simulink model "mysim22"  (R2021b)
settings: Solver=ode23t  StartTime=0.0  StopTime=70  RelTol=1e-3
libraries: fl_lib x15, nesl_utility x9, simulink x9, sh_lib x3, slpidlib x2
settings Model: Creator=camil  LastModifiedBy=camil

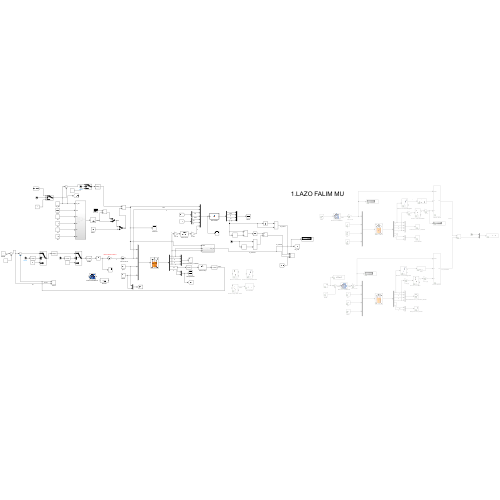
[thumbnail: Simulink's stored preview of the top-level diagram]
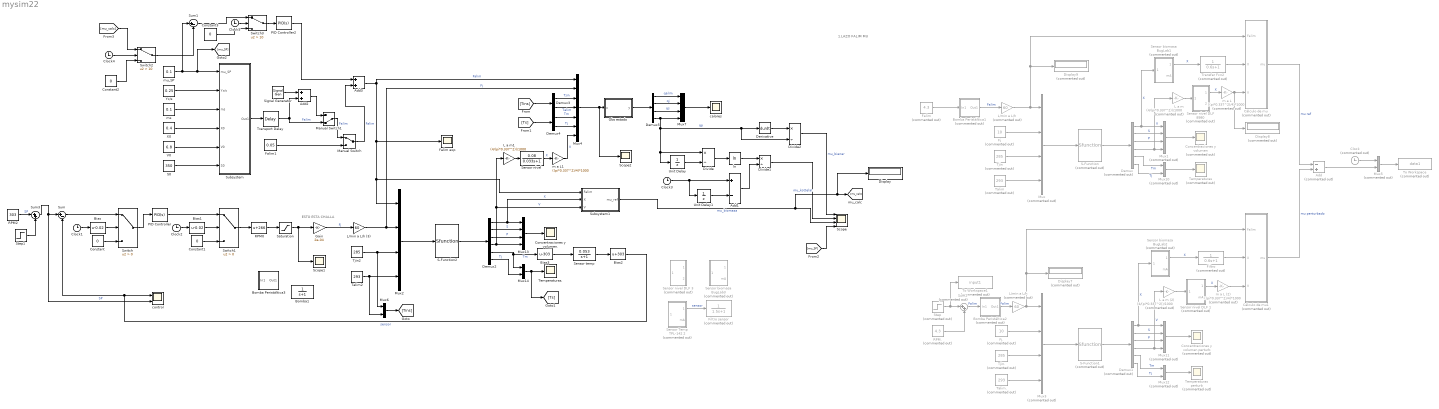
== system mysim22 ==
  note: ESTO ESTA CHALLA
  note: 1.LAZO FALIM MU
  Add : Sum  Commented=on  Inputs=-+
  Add1 : Sum  Inputs=+-
  Add2 : Sum
  Add3 : Sum
  Bias : Bias  Bias=-0.02
  Bias1 : Bias  Bias=-0.02
  Bias2 : Bias  Bias=303
  Bias3 : Bias  Bias=-303
  Bomba Peristáltica1 : Subsystem  Commented=on  mask{D=0.0002, MaxRPM=100, MaxLPM=0.036, OutP=0.14, FluidDens=997, KinemVisc=0.893e-6, BulkMod=2.2e+9}
      mask prompts: D "Displacement [L/rev]"; MaxRPM "RPM Máximas [RPM]"; MaxLPM "Caudal Máximo [L/min]"; OutP "Presión de Salida [MPa]"; FluidDens "Densidad del Fluido [kg/m^3]"; KinemVisc "Viscosidad Cinemática del Fluido [m^2/s]"; BulkMod "Modulo de Compresibilidad del Fluido [Pa]"
      mask help:
      | Simulación de una Bomba Peristáltica utilizando el paquete Simscape (puede entrar en el subsistema para ver en base a que bloques se construyó).
      |
      | El principal parámetro es el Displacement, que representa cuánto aumenta el flujo de la bomba medido en Litros por Minuto [L/min] según el aumento unitario de Revoluciones por Minuto [RPM].
      |
      | El input de este bloque es una fuente de revoluciones en unidades de RPM, el cual entrega un output de caudal en L/min.
      |
      | El valor del Displacement no puede superar su valor máximo según los parámetros entregados de la bomba.
      mask Display: image('bomba_peristaltica.jpg'); % Use "Edit Image" on toolstrip to change.
  Bomba Peristáltica2 : Subsystem  Commented=on  mask{D=0.0002, MaxRPM=100, MaxLPM=0.036, OutP=0.14, FluidDens=997, KinemVisc=0.893e-6, BulkMod=2.2e+9}
      mask prompts: D "Displacement [L/rev]"; MaxRPM "RPM Máximas [RPM]"; MaxLPM "Caudal Máximo [L/min]"; OutP "Presión de Salida [MPa]"; FluidDens "Densidad del Fluido [kg/m^3]"; KinemVisc "Viscosidad Cinemática del Fluido [m^2/s]"; BulkMod "Modulo de Compresibilidad del Fluido [Pa]"
      mask help:
      | Simulación de una Bomba Peristáltica utilizando el paquete Simscape (puede entrar en el subsistema para ver en base a que bloques se construyó).
      |
      | El principal parámetro es el Displacement, que representa cuánto aumenta el flujo de la bomba medido en Litros por Minuto [L/min] según el aumento unitario de Revoluciones por Minuto [RPM].
      |
      | El input de este bloque es una fuente de revoluciones en unidades de RPM, el cual entrega un output de caudal en L/min.
      |
      | El valor del Displacement no puede superar su valor máximo según los parámetros entregados de la bomba.
      mask Display: image('bomba_peristaltica.jpg'); % Use "Edit Image" on toolstrip to change.
  Bomba Peristáltica3 : Subsystem  mask{D=0.05, MaxRPM=330, MaxLPM=19.4, OutP=0.141, FluidDens=997, KinemVisc=0.893e-6, BulkMod=2.2e+9}
      mask prompts: D "Displacement [L/rev]"; MaxRPM "RPM Máximas [RPM]"; MaxLPM "Caudal Máximo [L/min]"; OutP "Presión de Salida [MPa]"; FluidDens "Densidad del Fluido [kg/m^3]"; KinemVisc "Viscosidad Cinemática del Fluido [m^2/s]"; BulkMod "Modulo de Compresibilidad del Fluido [Pa]"
      mask help:
      | Simulación de una Bomba Peristáltica utilizando el paquete Simscape (puede entrar en el subsistema para ver en base a que bloques se construyó).
      |
      | El principal parámetro es el Displacement, que representa cuánto aumenta el flujo de la bomba medido en Litros por Minuto [L/min] según el aumento unitario de Revoluciones por Minuto [RPM].
      |
      | El input de este bloque es una fuente de revoluciones en unidades de RPM, el cual entrega un output de caudal en L/min.
      |
      | El valor del Displacement no puede superar su valor máximo según los parámetros entregados de la bomba.
      mask Display: image('bomba_peristaltica.jpg'); % Use "Edit Image" on toolstrip to change.
  Bomba1 : TransferFcn  Denominator=[1 1]
  Clock : Clock  Commented=on
  Clock{1..5} (5 alike) : Clock
  Concentraciones y volumen : Scope  Commented=on
  Concentraciones y volumen perturb : Scope  Commented=on
  Concentraciones y volumen. : Scope
  Constant{,1..3} (4 alike) : Constant  Value=0
  Cálculo de mu : Subsystem  Commented=on
  Cálculo de mu1 : Subsystem  Commented=on
  Demux : Demux  Commented=on  Outputs=6
  Demux1 : Demux  Commented=on  Outputs=6
  Demux2 : Demux  Outputs=6
  Demux3 : Demux  Outputs=2
  Demux4 : Demux  Outputs=2
  Demux5 : Demux
  Derivative : Derivative
  Display : Display
  Display7 : Display  Commented=on
  Display8 : Display  Commented=on
  Display9 : Display  Commented=on
  Divide : Product  Inputs=*/
  Divide1 : Product  Inputs=*/
  Divide2 : Product  Inputs=*/
  Falim : Constant  Commented=on  Value=4.3
  Falim exp : Scope
  Falim1 : Constant  Value=0.05
  Filtro : TransferFcn  Commented=on  Denominator=[0.6 1]
  Filtro sensor : TransferFcn  Commented=on  Denominator=[1.5 1]
  Fj : Constant  Commented=on  Value=10
  Fj. : Constant  Commented=on  Value=10
  Gain : Gain  Gain=2e-04
  L a m : Gain  Commented=on  Gain=(4/(pi*0.337^2))/1000
  L a m (2) : Gain  Commented=on  Gain=(4/(pi*0.337^2))/1000
  L a m1 : Gain  Gain=(4/(pi*0.337^2))/1000
  L/min a L/h : Gain  Commented=on  Gain=60
  "L/min a L/h " : Gain  Commented=on  Gain=60
  L/min a L/h (3) : Gain  Gain=60
  Manual Switch : ManualSwitch
  Manual Switch1 : ManualSwitch  CurrentSetting=0
  Mux{,1,3,11} (4 alike) : Mux  Commented=on
  Mux10 : Mux  Commented=on  Inputs=2
  Mux12 : Mux  Commented=on  Inputs=2
  Mux13 : Mux
  Mux14 : Mux  Inputs=2
  Mux2 : Mux
  Mux4 : Mux  Inputs=7
  Mux5 : Mux  Commented=on  Inputs=2
  Mux6 : Mux  Inputs=2
  Mux7 : Mux
  Obs estado : MATLAB Function  TreatAsAtomicUnit=on
  PID Controller : slpidlib/PID Controller  Controller=PID  Form=Parallel  TimeDomain=Continuous-time  UseExternalTs=off  SampleTime=-1  IntegratorMethod=Forward Euler  FilterMethod=Forward Euler  ControllerParametersSource=internal  P=-2.038e+06  I=-6.635e+04  D=0  UseFilter=on  N=100  TunerSelectOption=Transfer Function Based (PID Tuner App)  InitialConditionSource=internal  InitialConditionForIntegrator=0  InitialConditionForFilter=0  DifferentiatorICPrevScaledInput=0  ExternalReset=none  TrackingMode=off  Kt=1  LimitOutput=off  SatLimitsSource=internal  UpperSaturationLimit=inf  LowerSaturationLimit=-inf  LinearizeAsGain=on  AntiWindupMode=none  Kb=1  RndMeth=Zero  POutMin=[]  POutMax=[]  IOutMin=[]  IOutMax=[]  DOutMin=[]  DOutMax=[]  NOutMin=[]  NOutMax=[]  SumOutMin=[]  SumOutMax=[]  SaturationOutMin=[]  SaturationOutMax=[]  PParamMin=[]  PParamMax=[]  IParamMin=[]  IParamMax=[]  DParamMin=[]  DParamMax=[]  NParamMin=[]  NParamMax=[]  KbParamMin=[]  KbParamMax=[]  KtParamMin=[]  KtParamMax=[]  KbOutMin=[]  KbOutMax=[]  KtOutMin=[]  KtOutMax=[]  IntegratorOutMin=[]  IntegratorOutMax=[]  FilterOutMin=[]  FilterOutMax=[]  SumI1OutMin=[]  SumI1OutMax=[]  SumI2OutMin=[]  SumI2OutMax=[]  SumI3OutMin=[]  SumI3OutMax=[]  SumI4OutMin=[]  SumI4OutMax=[]  SumDOutMin=[]  SumDOutMax=[]  DifferentiatorOutMin=[]  DifferentiatorOutMax=[]  FilterDiffOutCoefMin=[]  FilterDiffOutCoefMax=[]  ReciprocalOutMin=[]  ReciprocalOutMax=[]  SumDenOutMin=[]  SumDenOutMax=[]  SumNumOutMin=[]  SumNumOutMax=[]  DivideOutMin=[]  DivideOutMax=[]  UdiffTsProdOutMin=[]  UdiffTsProdOutMax=[]  NTsProdOutMin=[]  NTsProdOutMax=[]  UintegralTsProdOutMin=[]  UintegralTsProdOutMax=[]  UngainTsProdOutMin=[]  UngainTsProdOutMax=[]  IntegratorContinuousStateAttributes=''  IntegratorStateMustResolveToSignalObject=off  IntegratorRTWStateStorageClass=Auto  FilterContinuousStateAttributes=''  FilterStateMustResolveToSignalObject=off  FilterRTWStateStorageClass=Auto  ParallelPVariant=InternalParameters  IdealPVariant=Disabled  IVariant=InternalParameters  DVariant=InternalParameters  IntegratorVariant=Continuous  SatVariant=Disabled  AWVariant=Passthrough  PCopyVariant=Disabled  TRVariant=Disabled  FdbkBlocksVariant=Forward  IdealPFdbkVariant=Disabled  SatFdbkVariant=Disabled  DerivativeFilterVariant=ContFilter  NVariant=InternalParameters  NCopyVariant=Disabled  FilterICVariant=InternalICsFilter  IntegratorICVariant=InternalICs  ExternalResetVariant=Disabled  TRSumVariant=Passthrough  SumFdbkVariant=Disabled  SumVariant=Sum_PID  TsampFilterVariant=InternalTs  TsampNgainVariant=Passthrough  TsampIntegralVariant=Passthrough  ExternalSaturationOutDataTypeStr=Inherit: Same as second input
  PID Controller2 : slpidlib/PID Controller  Controller=PID  Form=Parallel  TimeDomain=Continuous-time  UseExternalTs=off  SampleTime=-1  IntegratorMethod=Forward Euler  FilterMethod=Forward Euler  ControllerParametersSource=internal  P=0.01  I=0.01  D=0.01  UseFilter=on  N=100  TunerSelectOption=Transfer Function Based (PID Tuner App)  InitialConditionSource=internal  InitialConditionForIntegrator=0  InitialConditionForFilter=0  DifferentiatorICPrevScaledInput=0  ExternalReset=none  TrackingMode=off  Kt=1  LimitOutput=off  SatLimitsSource=internal  UpperSaturationLimit=inf  LowerSaturationLimit=-inf  LinearizeAsGain=on  AntiWindupMode=none  Kb=1  POutMin=[]  POutMax=[]  IOutMin=[]  IOutMax=[]  DOutMin=[]  DOutMax=[]  NOutMin=[]  NOutMax=[]  SumOutMin=[]  SumOutMax=[]  SaturationOutMin=[]  SaturationOutMax=[]  PParamMin=[]  PParamMax=[]  IParamMin=[]  IParamMax=[]  DParamMin=[]  DParamMax=[]  NParamMin=[]  NParamMax=[]  KbParamMin=[]  KbParamMax=[]  KtParamMin=[]  KtParamMax=[]  KbOutMin=[]  KbOutMax=[]  KtOutMin=[]  KtOutMax=[]  IntegratorOutMin=[]  IntegratorOutMax=[]  FilterOutMin=[]  FilterOutMax=[]  SumI1OutMin=[]  SumI1OutMax=[]  SumI2OutMin=[]  SumI2OutMax=[]  SumI3OutMin=[]  SumI3OutMax=[]  SumI4OutMin=[]  SumI4OutMax=[]  SumDOutMin=[]  SumDOutMax=[]  DifferentiatorOutMin=[]  DifferentiatorOutMax=[]  FilterDiffOutCoefMin=[]  FilterDiffOutCoefMax=[]  ReciprocalOutMin=[]  ReciprocalOutMax=[]  SumDenOutMin=[]  SumDenOutMax=[]  SumNumOutMin=[]  SumNumOutMax=[]  DivideOutMin=[]  DivideOutMax=[]  UdiffTsProdOutMin=[]  UdiffTsProdOutMax=[]  NTsProdOutMin=[]  NTsProdOutMax=[]  UintegralTsProdOutMin=[]  UintegralTsProdOutMax=[]  UngainTsProdOutMin=[]  UngainTsProdOutMax=[]  IntegratorContinuousStateAttributes=''  IntegratorStateMustResolveToSignalObject=off  IntegratorRTWStateStorageClass=Auto  FilterContinuousStateAttributes=''  FilterStateMustResolveToSignalObject=off  FilterRTWStateStorageClass=Auto  ParallelPVariant=InternalParameters  IdealPVariant=Disabled  IVariant=InternalParameters  DVariant=InternalParameters  IntegratorVariant=Continuous  SatVariant=Disabled  AWVariant=Passthrough  PCopyVariant=Disabled  TRVariant=Disabled  FdbkBlocksVariant=Forward  IdealPFdbkVariant=Disabled  SatFdbkVariant=Disabled  DerivativeFilterVariant=ContFilter  NVariant=InternalParameters  NCopyVariant=Disabled  FilterICVariant=InternalICsFilter  IntegratorICVariant=InternalICs  ExternalResetVariant=Disabled  TRSumVariant=Passthrough  SumFdbkVariant=Disabled  SumVariant=Sum_PID  TsampFilterVariant=InternalTs  TsampNgainVariant=Passthrough  TsampIntegralVariant=Passthrough  ExternalSaturationOutDataTypeStr=Inherit: Same as second input
  RPM. : Constant  Commented=on  Value=4.3
  RPM0 : Bias  Bias=266
  RPM2 : Constant  Value=303
  S-Function : S-Function  Commented=on  FunctionName=Sfunction  SFunctionDeploymentMode=off  EnableBusSupport=off
      mask Display: image('bioreactor.png'); % Use "Edit Image" on toolstrip to change.
  S-Function1 : S-Function  Commented=on  FunctionName=Sfunction  SFunctionDeploymentMode=off  EnableBusSupport=off
      mask Display: image('bioreactor.png'); % Use "Edit Image" on toolstrip to change.
  S-Function2 : S-Function  FunctionName=Sfunction  SFunctionDeploymentMode=off  EnableBusSupport=off
      mask Display: image('bioreactor.png'); % Use "Edit Image" on toolstrip to change.
  S0 : Constant  Value=350
  Saturation : Saturate  UpperLimit=1.5  LowerLimit=0
  Scope : Scope  NumInputPorts=4
  Scope1 : Scope
  Scope2 : Scope
  Sensor Temp TPL-142 2 : Subsystem  Commented=on  mask{To=0.1733, d=0, DS=0.075, Ks=0.053, Tau=1.733, yo=0.003, Vi=300}
      mask prompts: To "Tiempo de muestreo (s)"; d "Retardo (s)"; DS "Desviacion estandar (pH)"; Ks "Sensibilidad (mA/pH)"; Tau "Constante de tiempo (s)"; yo "Sesgo (pH)"; Vi "Valor inicial (pH)"
      mask init:
      | NP=To*DS*DS;
      mask Display: image(imread('sensor_temperatura.jpg'))
  Sensor biomasa BugLab1 : Subsystem  Commented=on  mask{To=0.01, d=0, DS=0.075, Ks=0.08, Tau=0.0067, yo=0, Vi=0}
      mask prompts: To "Tiempo de muestreo (s)"; d "Retardo (s)"; DS "Desviacion estandar (g/L)"; Ks "Sensibilidad (mA/g/L)"; Tau "Constante de tiempo (s)"; yo "Sesgo (g/L)"; Vi "Valor inicial (g/L)"
      mask init:
      | NP=To*DS*DS;
      mask Display: image(imread('sensor_biomasa.png'))
  Sensor biomasa BugLab2 : Subsystem  Commented=on  mask{To=0.01, d=0, DS=0.075, Ks=0.08, Tau=0.0067, yo=0, Vi=0}
      mask prompts: To "Tiempo de muestreo (s)"; d "Retardo (s)"; DS "Desviacion estandar (g/L)"; Ks "Sensibilidad (mA/g/L)"; Tau "Constante de tiempo (s)"; yo "Sesgo (g/L)"; Vi "Valor inicial (g/L)"
      mask init:
      | NP=To*DS*DS;
      mask Display: image(imread('sensor_biomasa.png'))
  Sensor biomasa BugLab3 : Subsystem  Commented=on  mask{To=0.01, d=0, DS=0.075, Ks=0.08, Tau=0.0067, yo=0, Vi=0}
      mask prompts: To "Tiempo de muestreo (s)"; d "Retardo (s)"; DS "Desviacion estandar (g/L)"; Ks "Sensibilidad (mA/g/L)"; Tau "Constante de tiempo (s)"; yo "Sesgo (g/L)"; Vi "Valor inicial (g/L)"
      mask init:
      | NP=To*DS*DS;
      mask Display: image(imread('sensor_biomasa.png'))
  Sensor nivel : TransferFcn  Numerator=[0.08]  Denominator=[0.033 1]
  Sensor nivel DLF 1 : Subsystem  Commented=on  mask{To=0.1, d=0, DS=0.005, Ks=0.08, Tau=0.033, yo=0, Vi=0}
      mask prompts: To "Tiempo de muestreo (s)"; d "Retardo (s)"; DS "Desviacion estandar (g/L)"; Ks "Sensibilidad (mA/g/L)"; Tau "Constante de tiempo (s)"; yo "Sesgo (g/L)"; Vi "Valor inicial (g/L)"
      mask init:
      | NP=To*DS*DS;
      mask Display: image(imread('sensor_nivel.jpg'))
  Sensor nivel DLF 3 : Subsystem  Commented=on  mask{To=0.1, d=0, DS=0.005, Ks=0.08, Tau=0.033, yo=0, Vi=0}
      mask prompts: To "Tiempo de muestreo (s)"; d "Retardo (s)"; DS "Desviacion estandar (g/L)"; Ks "Sensibilidad (mA/g/L)"; Tau "Constante de tiempo (s)"; yo "Sesgo (g/L)"; Vi "Valor inicial (g/L)"
      mask init:
      | NP=To*DS*DS;
      mask Display: image(imread('sensor_nivel.jpg'))
  Sensor nivel DLF 8980 : Subsystem  Commented=on  mask{To=0.1, d=0, DS=0.005, Ks=0.08, Tau=0.033, yo=0, Vi=0}
      mask prompts: To "Tiempo de muestreo (s)"; d "Retardo (s)"; DS "Desviacion estandar (g/L)"; Ks "Sensibilidad (mA/g/L)"; Tau "Constante de tiempo (s)"; yo "Sesgo (g/L)"; Vi "Valor inicial (g/L)"
      mask init:
      | NP=To*DS*DS;
      mask Display: image(imread('sensor_nivel.jpg'))
  Sensor temp : TransferFcn  Numerator=[0.053]  Denominator=[1 1]
  Signal Generator : SignalGenerator  Frequency=0.5  Units=rad/sec
  Step : Step  Commented=on  Time=25  After=0.4  SampleTime=0
  Step1 : Step  Time=10  After=0  SampleTime=0
  Subsystem : Subsystem
  Subsystem1 : Subsystem
  Sum : Sum  Inputs=|+-
  Sum1 : Sum  Inputs=|+-
  Sum2 : Sum  Commented=on  Inputs=|++
  Sum3 : Sum  Inputs=|++
  Switch : Switch  Criteria=u2 > Threshold
  Switch1 : Switch  Criteria=u2 > Threshold
  Switch2 : Switch  Criteria=u2 > Threshold  Threshold=10
  Switch3 : Switch  Criteria=u2 > Threshold  Threshold=10
  Talim : Constant  Commented=on  Value=293
  Talim. : Constant  Commented=on  Value=293
  Talim2 : Constant  Value=293
  Temperaturas : Scope  Commented=on
  Temperaturas perturb : Scope  Commented=on
  Temperaturas. : Scope
  Tjin : Constant  Commented=on  Value=285
  Tjin. : Constant  Commented=on  Value=285
  Tjin2 : Constant  Value=285
  To Workspace : ToWorkspace  Commented=on  VariableName=data1  SampleTime=1
  To Workspace1 : ToWorkspace  Commented=on  VariableName=input1  SampleTime=1
  Transfer Fcn2 : TransferFcn  Commented=on  Denominator=[0.6 1]
  Transport Delay : TransportDelay
  Unit Delay : UnitDelay  SampleTime=-1  HasFrameUpgradeWarning=on
  Unit Delay1 : UnitDelay  SampleTime=-1  HasFrameUpgradeWarning=on
  V0 : Constant  Value=6.8
  X0 : Constant  Value=0.4
  Yx/s : Constant  Value=0.25
  calores : Scope
  control : Scope  NumInputPorts=2
  ln : Math  Operator=log  SaturateOnIntegerOverflow=on
  m a L : Gain  Commented=on  Gain=((pi*0.337^2)/4)*1000
  m a L (2) : Gain  Commented=on  Gain=((pi*0.337^2)/4)*1000
  m a L1 : Gain  Gain=((pi*0.337^2)/4)*1000
  ms : Constant  Value=0.1
  mu_SP : Constant  Value=0.1
  wires:
  Fj/1 -> Mux/2
  Mux/1 -> S-Function/1
  S-Function/1 -> Demux/1
  Demux/2 -> Mux1/2  "S"
  Demux/3 -> Mux1/3  "P"
  Mux1/1 -> Concentraciones y volumen/1
  Demux/4 -> L a m/1, Mux1/4  "V"
  Demux/5 -> Mux10/1  "Tm"
  Demux/6 -> Mux10/2  "Tj"
  Talim/1 -> Mux/4
  Tjin/1 -> Mux/3
  Demux1/2 -> Mux11/2  "S"
  Demux1/3 -> Mux11/3  "P"
  Talim./1 -> Mux3/4
  Demux1/5 -> Mux12/1  "Tm"
  Demux1/6 -> Mux12/2  "Tj"
  S-Function1/1 -> Demux1/1
  Mux3/1 -> S-Function1/1
  Tjin./1 -> Mux3/3
  Fj./1 -> Mux3/2
  RPM./1 -> Sum2/2
  Step/1 -> To Workspace1/1, Sum2/1
  Mux5/1 -> To Workspace/1
  Clock/1 -> Mux5/1
  Add/1 -> Mux5/2
  Demux1/4 -> Mux11/4, L a m (2)/1  "V"
  Demux1/1 -> Mux11/1, Sensor biomasa BugLab2/1(señal medida)  "X"
  Mux13/1 -> Concentraciones y volumen./1
  Demux2/3 -> Mux13/3  "P"
  Demux2/1 -> Subsystem1/2(X), Mux13/1  "X"
  Demux2/2 -> Mux13/2  "S"
  Demux2/5 -> Bias3/1, Mux14/1  "Tm"
  S-Function2/1 -> Demux2/1
  Mux2/1 -> S-Function2/1
  Demux2/6 -> Mux14/2  "Tj"
  Demux2/4 -> Mux13/4, L a m1/1, Subsystem1/3(V)  "V"
  Demux/1 -> Sensor biomasa BugLab1/1(señal medida), Mux1/1  "X"
  Falim/1 -> Bomba Peristáltica1/1(In1)
  Sum3/1 -> control/2, Sum/1  "SP"
  L a m/1 -> Sensor nivel DLF 8980/1(señal medida)
  Sensor nivel DLF 8980/1(biomasa) -> m a L/1  "X"
  Sensor nivel DLF 1/1(biomasa) -> m a L (2)/1  "X"
  L a m (2)/1 -> Sensor nivel DLF 1/1(señal medida)
  Sum2/1 -> Bomba Peristáltica2/1(In1)  "Falim"
  Mux10/1 -> Temperaturas/1
  m a L/1 -> Display8/1, Cálculo de mu/3(V)
  Sensor biomasa BugLab1/1(biomasa) -> Transfer Fcn2/1  "X"
  Cálculo de mu/1(mu) -> Add/1  "mu ref"
  m a L (2)/1 -> Cálculo de mu1/3(V)
  Cálculo de mu1/1(mu) -> Add/2  "mu perturbado"
  Sensor biomasa BugLab2/1(biomasa) -> Filtro/1  "X"
  Mux14/1 -> [Ts], Temperaturas./1
  Gain/1 -> L/min a L/h (3)/1  "Fj"
  L/min a L/h (3)/1 -> Mux2/2, Mux4/2  "Fj"
  Bomba Peristáltica1/1(Out1) -> "L/min a L/h "/1  "Falim"
  Bomba Peristáltica2/1(Out1) -> L/min a L/h/1  "Falim"
  "L/min a L/h "/1 -> Cálculo de mu/1(Falim), Display9/1, Mux/1
  L/min a L/h/1 -> Cálculo de mu1/1(Falim), Display7/1, Mux3/1
  Transfer Fcn2/1 -> Cálculo de mu/2(X)
  Filtro/1 -> Cálculo de mu1/2(X)
  Bias2/1 -> Sum/2, control/1  "sensor"
  Mux12/1 -> Temperaturas perturb/1
  Mux11/1 -> Concentraciones y volumen perturb/1
  Saturation/1 -> Gain/1, Scope1/1
  Sum/1 -> Switch/1
  mu_SP/1 -> [mu_SP], Subsystem/1(mu_SP), Sum1/1
  Yx/s/1 -> Subsystem/2(Yx/s)
  ms/1 -> Subsystem/3(ms)
  X0/1 -> Subsystem/4(X0)
  V0/1 -> Subsystem/5(V0)
  Subsystem/1(Out1) -> Transport Delay/1
  S0/1 -> Subsystem/6(S0)
  Talim2/1 -> Mux6/2, Mux2/4
  Tjin2/1 -> Mux2/3, Mux6/1
  Mux4/1 -> Scope2/1, Obs estado/1(u)
  Mux6/1 -> [Tins]
  Demux3/1 -> Mux4/3  "Tjin"
  Demux3/2 -> Mux4/4  "Talim"
  [Tins] -> Demux3/1
  [Ts] -> Demux4/1
  Demux4/1 -> Mux4/5  "Tm"
  Demux4/2 -> Mux4/6  "Tj"
  Obs estado/1(y) -> Demux5/1
  Mux7/1 -> calores/1
  Demux5/1 -> Mux7/1  "qalim"
  Demux5/2 -> Mux7/2  "qj"
  Demux5/3 -> Mux7/3  "qs"
  Demux5/4 -> Unit Delay/1, Divide/1, Divide2/2, Derivative/1, Mux7/4  "qp"
  Falim1/1 -> Manual Switch/2
  Transport Delay/1 -> Manual Switch1/2, Add2/2  "Falim"
  Add3/1 -> Mux4/1, Falim exp/1, Subsystem1/1(Falim), Mux2/1  "Falim"
  Switch/1 -> PID Controller/1
  Constant/1 -> Switch/3
  Clock1/1 -> Bias/1
  Bias/1 -> Switch/2
  Clock2/1 -> Bias1/1
  Bias1/1 -> Switch1/2
  Constant1/1 -> Switch1/3
  Switch1/1 -> RPM0/1
  PID Controller/1 -> Switch1/1
  RPM0/1 -> Saturation/1
  Bias3/1 -> Sensor temp/1
  Sensor temp/1 -> Bias2/1
  Sensor Temp TPL-142 2/1(biomasa) -> Filtro sensor/1  "sensor"
  Sensor nivel/1 -> m a L1/1  "X"
  L a m1/1 -> Sensor nivel/1
  m a L1/1 -> Mux4/7  "V"
  Unit Delay/1 -> Divide/2
  Divide/1 -> ln/1
  Clock3/1 -> Unit Delay1/1, Add1/1
  Unit Delay1/1 -> Add1/2
  ln/1 -> Divide1/1
  Add1/1 -> Divide1/2
  Divide1/1 -> Scope/2  "mu_kottelat"
  Subsystem1/1(mu_ref) -> Display/1, [mu_calc], Scope/3  "mu_biomasa"
  Derivative/1 -> Divide2/1
  Divide2/1 -> Scope/1  "mu_biener"
  Signal Generator/1 -> Add2/1
  Add2/1 -> Manual Switch1/1
  [mu_SP] -> Scope/4
  Manual Switch1/1 -> Manual Switch/1  "Falim"
  [mu_calc] -> Switch2/1
  Sum1/1 -> Switch3/1
  Manual Switch/1 -> Add3/2  "Falim"
  PID Controller2/1 -> Add3/1
  RPM2/1 -> Sum3/1  "SP"
  Step1/1 -> Sum3/2
  Switch2/1 -> Sum1/2
  Clock4/1 -> Switch2/2
  Constant2/1 -> Switch2/3
  Constant3/1 -> Switch3/3
  Switch3/1 -> PID Controller2/1
  Clock5/1 -> Switch3/2

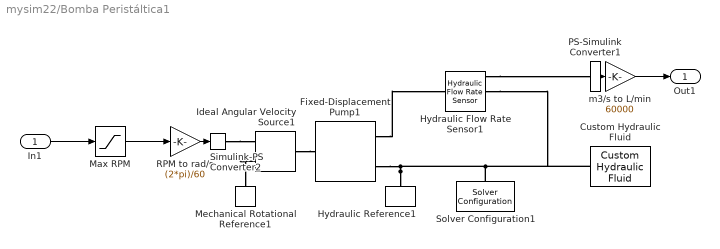
== system mysim22/Bomba Peristáltica1 ==
  In1 : Inport
  Custom Hydraulic Fluid : fl_lib/Hydraulic/Hydraulic Utilities/Custom Hydraulic Fluid  density=FluidDens kg/m^3  viscosity_kin=KinemVisc m^2/s  bulk=BulkMod Pa  alpha=0  range_error=2
      settings: SourceProductBaseCode=SS  InternalSimscapePortConfiguration="{\"Bottom\":[],\"Left\":[],\"Right\":[{\"id\":\"G\",\"label\":\"\",\"type\":\"foundation.hydraulic.hydraulic\"}],\"Top\":[]}"
  Fixed-Displacement Pump1 : sh_lib/Pumps and Motors/Fixed-Displacement Pump  D=D l/rev  loss_spec=1  w_nominal=MaxRPM rpm  pr_nominal=OutP MPa  visc_nominal=KinemVisc m^2/s  dens_nominal=FluidDens kg/m^3  efficiency_vol=1  no_load_torque=0 N*m  torque_pressure_coeff=0 N*m/Pa  p_diff_eff_TLU=[100000, 1000000, 2000000] Pa  omega_eff_TLU=[25, 50, 100, 200, 300, 400] rad/s  vol_eff_TLU=[.816, .908, .954, .977, .981, .984; .325, .663, .831, .916, .925, .946; .137, .568, .78, .892, .893, .91]  mech_eff_TLU=[.996, .996, .996, .996, .996, .996; .988, .989, .989, .989, .989, .99; .981, .981, .982, .982, .983, .984]  p_diff_loss_TLU=[100000, 1000000, 2000000] Pa  omega_loss_TLU=[25, 50, 100, 200, 300, 400] rad/s  vol_loss_TLU=[.023, .023, .023, .023, .0285, .032; .0844, .0842, .0845, .084, .1125, .108; .1079, .108, .11, .108, .1605, .18] * 1e-3 m^3/s  mech_loss_TLU=[.002, .002, .002, .002, .002, .002; .0607, .0556, .0556, .0556, .0556, .0505; .1937, .1937, .1833, .1833, .1729, .1626] N*m  pressure_threshold=1e5 Pa  omega_threshold=10 rad/s  quadrant_check=0  pressure_check=0  min_valid_pressure=0 Pa  vol_eff_min=1e-3  vol_eff_max=1  mech_eff_min=1e-3  mech_eff_max=1
      settings: SourceProductBaseCode=SH  InternalSimscapePortConfiguration="{\"Bottom\":[],\"Left\":[{\"id\":\"S\",\"label\":\"S\",\"type\":\"foundation.mechanical.rotational.rotational\"}],\"Right\":[{\"id\":\"P\",\"label\":\"P\",\"type\":\"foundation.hydraulic.hydraulic\"},{\"id\":\"T\",\"label\":\"T\",\"type\":\"foundation.hydraulic.hydraulic\"}],\"Top\":[]}"
  Hydraulic Flow Rate Sensor1 : fl_lib/Hydraulic/Hydraulic Sensors/Hydraulic Flow Rate Sensor
  Hydraulic Reference1 : fl_lib/Hydraulic/Hydraulic Elements/Hydraulic Reference
  Ideal Angular Velocity Source1 : fl_lib/Mechanical/Mechanical Sources/Ideal Angular Velocity Source
  Max RPM : Saturate  UpperLimit=600  LowerLimit=0
  Mechanical Rotational Reference1 : fl_lib/Mechanical/Rotational Elements/Mechanical Rotational Reference
  PS-Simulink Converter1 : nesl_utility/PS-Simulink Converter  PhysicalDomain=network_engine_domain  SubClassName=ps_output  LeftPortType=input  RightPortType=output  PseudoPeriodic=off  Frequencies=[]  Unit=inherit  AffineConversion=off
      settings: SourceProductBaseCode=PW,SS
  RPM to rad/s : Gain  Gain=(2*pi)/60
  Simulink-PS Converter2 : nesl_utility/Simulink-PS Converter  PhysicalDomain=network_engine_domain  SubClassName=ps_input  LeftPortType=input  RightPortType=output  PseudoPeriodic=off  Frequencies=[]  NoiseDistribution=none  NoiseParameters=[]  Unit=1  AffineConversion=off  FilteringAndDerivatives=provide  SimscapeFilterOrder=1  InputFilterTimeConstant=0.001  UdotUserProvided=0
      settings: SourceProductBaseCode=PW,SS
  Solver Configuration1 : nesl_utility/Solver Configuration  PhysicalDomain=network_engine_domain  SubClassName=solver  LeftPortType=input  RightPortType=generic  Tones=[]  Harmonics=[]  SimulateNoise=off  Profile=off  UseLocalSampling=off  EnableSwitchedLinearOptims=on  FrequencyDomain=off  UseCCode=off  RelTol=0.001  AbsTol=1e-06  MinStep=1e-09  ToWorkspace=off  RevertToSquareIcSolve=off  NumHomotopyIterations=100  PhasorMode=off  PhasorModeNumHarmonics=1  DoDC=off  ResidualTolerance=1e-09  UseLocalSolver=off  LocalSolverChoice=NE_BACKWARD_EULER_ADVANCER  LocalSolverSampleTime=0.001  DoFixedCost=off  MaxNonlinIter=3  MaxModeIter=2  ComputeImpulses=off  ImpulseIterations=2  LinearAlgebra=auto  EquationFormulation=NE_TIME_EF  DelaysMemoryBudget=1024  AutomaticFiltering=on  FilteringTimeConstant=0.001  PartitionStorageMethod=AS_NEEDED  PartitionMemoryBudget=1024  PartitionMethod=ROBUST
      settings: SourceProductBaseCode=PW,SS
  m3/s to L/min : Gain  Gain=60000
  Out1 : Outport
  wires:
  RPM to rad/s/1 -> Simulink-PS Converter2/1
  PS-Simulink Converter1/1 -> m3/s to L/min/1
  In1/1 -> Max RPM/1
  m3/s to L/min/1 -> Out1/1
  Max RPM/1 -> RPM to rad/s/1
  connections:
  Hydraulic Reference1/LConn1 -- Custom Hydraulic Fluid/RConn1 -- Hydraulic Flow Rate Sensor1/RConn2 -- Solver Configuration1/RConn1 -- Fixed-Displacement Pump1/RConn2
  Simulink-PS Converter2/RConn1 -- Ideal Angular Velocity Source1/RConn1
  Ideal Angular Velocity Source1/RConn2 -- Mechanical Rotational Reference1/LConn1
  Hydraulic Flow Rate Sensor1/RConn1 -- PS-Simulink Converter1/LConn1
  Fixed-Displacement Pump1/RConn1 -- Hydraulic Flow Rate Sensor1/LConn1
  Ideal Angular Velocity Source1/LConn1 -- Fixed-Displacement Pump1/LConn1

== system mysim22/Bomba Peristáltica2 ==
  In1 : Inport
  Custom Hydraulic Fluid : fl_lib/Hydraulic/Hydraulic Utilities/Custom Hydraulic Fluid  density=FluidDens kg/m^3  viscosity_kin=KinemVisc m^2/s  bulk=BulkMod Pa  alpha=0  range_error=2
      settings: SourceProductBaseCode=SS  InternalSimscapePortConfiguration="{\"Bottom\":[],\"Left\":[],\"Right\":[{\"id\":\"G\",\"label\":\"\",\"type\":\"foundation.hydraulic.hydraulic\"}],\"Top\":[]}"
  Fixed-Displacement Pump1 : sh_lib/Pumps and Motors/Fixed-Displacement Pump  D=D l/rev  loss_spec=1  w_nominal=MaxRPM rpm  pr_nominal=OutP MPa  visc_nominal=KinemVisc m^2/s  dens_nominal=FluidDens kg/m^3  efficiency_vol=1  no_load_torque=0 N*m  torque_pressure_coeff=0 N*m/Pa  p_diff_eff_TLU=[100000, 1000000, 2000000] Pa  omega_eff_TLU=[25, 50, 100, 200, 300, 400] rad/s  vol_eff_TLU=[.816, .908, .954, .977, .981, .984; .325, .663, .831, .916, .925, .946; .137, .568, .78, .892, .893, .91]  mech_eff_TLU=[.996, .996, .996, .996, .996, .996; .988, .989, .989, .989, .989, .99; .981, .981, .982, .982, .983, .984]  p_diff_loss_TLU=[100000, 1000000, 2000000] Pa  omega_loss_TLU=[25, 50, 100, 200, 300, 400] rad/s  vol_loss_TLU=[.023, .023, .023, .023, .0285, .032; .0844, .0842, .0845, .084, .1125, .108; .1079, .108, .11, .108, .1605, .18] * 1e-3 m^3/s  mech_loss_TLU=[.002, .002, .002, .002, .002, .002; .0607, .0556, .0556, .0556, .0556, .0505; .1937, .1937, .1833, .1833, .1729, .1626] N*m  pressure_threshold=1e5 Pa  omega_threshold=10 rad/s  quadrant_check=0  pressure_check=0  min_valid_pressure=0 Pa  vol_eff_min=1e-3  vol_eff_max=1  mech_eff_min=1e-3  mech_eff_max=1
      settings: SourceProductBaseCode=SH  InternalSimscapePortConfiguration="{\"Bottom\":[],\"Left\":[{\"id\":\"S\",\"label\":\"S\",\"type\":\"foundation.mechanical.rotational.rotational\"}],\"Right\":[{\"id\":\"P\",\"label\":\"P\",\"type\":\"foundation.hydraulic.hydraulic\"},{\"id\":\"T\",\"label\":\"T\",\"type\":\"foundation.hydraulic.hydraulic\"}],\"Top\":[]}"
  Hydraulic Flow Rate Sensor1 : fl_lib/Hydraulic/Hydraulic Sensors/Hydraulic Flow Rate Sensor
  Hydraulic Reference1 : fl_lib/Hydraulic/Hydraulic Elements/Hydraulic Reference
  Ideal Angular Velocity Source1 : fl_lib/Mechanical/Mechanical Sources/Ideal Angular Velocity Source
  Max RPM : Saturate  UpperLimit=600  LowerLimit=0
  Mechanical Rotational Reference1 : fl_lib/Mechanical/Rotational Elements/Mechanical Rotational Reference
  PS-Simulink Converter1 : nesl_utility/PS-Simulink Converter  PhysicalDomain=network_engine_domain  SubClassName=ps_output  LeftPortType=input  RightPortType=output  PseudoPeriodic=off  Frequencies=[]  Unit=inherit  AffineConversion=off
      settings: SourceProductBaseCode=PW,SS
  RPM to rad/s : Gain  Gain=(2*pi)/60
  Simulink-PS Converter2 : nesl_utility/Simulink-PS Converter  PhysicalDomain=network_engine_domain  SubClassName=ps_input  LeftPortType=input  RightPortType=output  PseudoPeriodic=off  Frequencies=[]  NoiseDistribution=none  NoiseParameters=[]  Unit=1  AffineConversion=off  FilteringAndDerivatives=provide  SimscapeFilterOrder=1  InputFilterTimeConstant=0.001  UdotUserProvided=0
      settings: SourceProductBaseCode=PW,SS
  Solver Configuration1 : nesl_utility/Solver Configuration  PhysicalDomain=network_engine_domain  SubClassName=solver  LeftPortType=input  RightPortType=generic  Tones=[]  Harmonics=[]  SimulateNoise=off  Profile=off  UseLocalSampling=off  EnableSwitchedLinearOptims=on  FrequencyDomain=off  UseCCode=off  RelTol=0.001  AbsTol=1e-06  MinStep=1e-09  ToWorkspace=off  RevertToSquareIcSolve=off  NumHomotopyIterations=100  PhasorMode=off  PhasorModeNumHarmonics=1  DoDC=off  ResidualTolerance=1e-09  UseLocalSolver=off  LocalSolverChoice=NE_BACKWARD_EULER_ADVANCER  LocalSolverSampleTime=0.001  DoFixedCost=off  MaxNonlinIter=3  MaxModeIter=2  ComputeImpulses=off  ImpulseIterations=2  LinearAlgebra=auto  EquationFormulation=NE_TIME_EF  DelaysMemoryBudget=1024  AutomaticFiltering=on  FilteringTimeConstant=0.001  PartitionStorageMethod=AS_NEEDED  PartitionMemoryBudget=1024  PartitionMethod=ROBUST
      settings: SourceProductBaseCode=PW,SS
  m3/s to L/min : Gain  Gain=60000
  Out1 : Outport
  wires:
  RPM to rad/s/1 -> Simulink-PS Converter2/1
  PS-Simulink Converter1/1 -> m3/s to L/min/1
  In1/1 -> Max RPM/1
  m3/s to L/min/1 -> Out1/1
  Max RPM/1 -> RPM to rad/s/1
  connections:
  Hydraulic Reference1/LConn1 -- Custom Hydraulic Fluid/RConn1 -- Hydraulic Flow Rate Sensor1/RConn2 -- Solver Configuration1/RConn1 -- Fixed-Displacement Pump1/RConn2
  Simulink-PS Converter2/RConn1 -- Ideal Angular Velocity Source1/RConn1
  Ideal Angular Velocity Source1/RConn2 -- Mechanical Rotational Reference1/LConn1
  Hydraulic Flow Rate Sensor1/RConn1 -- PS-Simulink Converter1/LConn1
  Fixed-Displacement Pump1/RConn1 -- Hydraulic Flow Rate Sensor1/LConn1
  Ideal Angular Velocity Source1/LConn1 -- Fixed-Displacement Pump1/LConn1

== system mysim22/Bomba Peristáltica3 ==
  In1 : Inport
  Custom Hydraulic Fluid : fl_lib/Hydraulic/Hydraulic Utilities/Custom Hydraulic Fluid  density=FluidDens kg/m^3  viscosity_kin=KinemVisc m^2/s  bulk=BulkMod Pa  alpha=0  range_error=2
      settings: SourceProductBaseCode=SS  InternalSimscapePortConfiguration="{\"Bottom\":[],\"Left\":[],\"Right\":[{\"id\":\"G\",\"label\":\"\",\"type\":\"foundation.hydraulic.hydraulic\"}],\"Top\":[]}"
  Fixed-Displacement Pump1 : sh_lib/Pumps and Motors/Fixed-Displacement Pump  D=D l/rev  loss_spec=1  w_nominal=MaxRPM rpm  pr_nominal=OutP MPa  visc_nominal=KinemVisc m^2/s  dens_nominal=FluidDens kg/m^3  efficiency_vol=1  no_load_torque=0 N*m  torque_pressure_coeff=0 N*m/Pa  p_diff_eff_TLU=[100000, 1000000, 2000000] Pa  omega_eff_TLU=[25, 50, 100, 200, 300, 400] rad/s  vol_eff_TLU=[.816, .908, .954, .977, .981, .984; .325, .663, .831, .916, .925, .946; .137, .568, .78, .892, .893, .91]  mech_eff_TLU=[.996, .996, .996, .996, .996, .996; .988, .989, .989, .989, .989, .99; .981, .981, .982, .982, .983, .984]  p_diff_loss_TLU=[100000, 1000000, 2000000] Pa  omega_loss_TLU=[25, 50, 100, 200, 300, 400] rad/s  vol_loss_TLU=[.023, .023, .023, .023, .0285, .032; .0844, .0842, .0845, .084, .1125, .108; .1079, .108, .11, .108, .1605, .18] * 1e-3 m^3/s  mech_loss_TLU=[.002, .002, .002, .002, .002, .002; .0607, .0556, .0556, .0556, .0556, .0505; .1937, .1937, .1833, .1833, .1729, .1626] N*m  pressure_threshold=1e5 Pa  omega_threshold=10 rad/s  quadrant_check=0  pressure_check=0  min_valid_pressure=0 Pa  vol_eff_min=1e-3  vol_eff_max=1  mech_eff_min=1e-3  mech_eff_max=1
      settings: SourceProductBaseCode=SH  InternalSimscapePortConfiguration="{\"Bottom\":[],\"Left\":[{\"id\":\"S\",\"label\":\"S\",\"type\":\"foundation.mechanical.rotational.rotational\"}],\"Right\":[{\"id\":\"P\",\"label\":\"P\",\"type\":\"foundation.hydraulic.hydraulic\"},{\"id\":\"T\",\"label\":\"T\",\"type\":\"foundation.hydraulic.hydraulic\"}],\"Top\":[]}"
  Hydraulic Flow Rate Sensor1 : fl_lib/Hydraulic/Hydraulic Sensors/Hydraulic Flow Rate Sensor
  Hydraulic Reference1 : fl_lib/Hydraulic/Hydraulic Elements/Hydraulic Reference
  Ideal Angular Velocity Source1 : fl_lib/Mechanical/Mechanical Sources/Ideal Angular Velocity Source
  Max RPM : Saturate  UpperLimit=600  LowerLimit=0
  Mechanical Rotational Reference1 : fl_lib/Mechanical/Rotational Elements/Mechanical Rotational Reference
  PS-Simulink Converter1 : nesl_utility/PS-Simulink Converter  PhysicalDomain=network_engine_domain  SubClassName=ps_output  LeftPortType=input  RightPortType=output  PseudoPeriodic=off  Frequencies=[]  Unit=inherit  AffineConversion=off
      settings: SourceProductBaseCode=PW,SS
  RPM to rad/s : Gain  Gain=(2*pi)/60
  Simulink-PS Converter2 : nesl_utility/Simulink-PS Converter  PhysicalDomain=network_engine_domain  SubClassName=ps_input  LeftPortType=input  RightPortType=output  PseudoPeriodic=off  Frequencies=[]  NoiseDistribution=none  NoiseParameters=[]  Unit=1  AffineConversion=off  FilteringAndDerivatives=provide  SimscapeFilterOrder=1  InputFilterTimeConstant=0.001  UdotUserProvided=0
      settings: SourceProductBaseCode=PW,SS
  Solver Configuration1 : nesl_utility/Solver Configuration  PhysicalDomain=network_engine_domain  SubClassName=solver  LeftPortType=input  RightPortType=generic  Tones=[]  Harmonics=[]  SimulateNoise=off  Profile=off  UseLocalSampling=off  EnableSwitchedLinearOptims=on  FrequencyDomain=off  UseCCode=off  RelTol=0.001  AbsTol=1e-06  MinStep=1e-09  ToWorkspace=off  RevertToSquareIcSolve=off  NumHomotopyIterations=100  PhasorMode=off  PhasorModeNumHarmonics=1  DoDC=off  ResidualTolerance=1e-09  UseLocalSolver=off  LocalSolverChoice=NE_BACKWARD_EULER_ADVANCER  LocalSolverSampleTime=0.001  DoFixedCost=off  MaxNonlinIter=3  MaxModeIter=2  ComputeImpulses=off  ImpulseIterations=2  LinearAlgebra=auto  EquationFormulation=NE_TIME_EF  DelaysMemoryBudget=1024  AutomaticFiltering=on  FilteringTimeConstant=0.001  PartitionStorageMethod=AS_NEEDED  PartitionMemoryBudget=1024  PartitionMethod=ROBUST
      settings: SourceProductBaseCode=PW,SS
  m3/s to L/min : Gain  Gain=60000
  Out1 : Outport
  wires:
  RPM to rad/s/1 -> Simulink-PS Converter2/1
  PS-Simulink Converter1/1 -> m3/s to L/min/1
  In1/1 -> Max RPM/1
  m3/s to L/min/1 -> Out1/1
  Max RPM/1 -> RPM to rad/s/1
  connections:
  Hydraulic Reference1/LConn1 -- Custom Hydraulic Fluid/RConn1 -- Hydraulic Flow Rate Sensor1/RConn2 -- Solver Configuration1/RConn1 -- Fixed-Displacement Pump1/RConn2
  Simulink-PS Converter2/RConn1 -- Ideal Angular Velocity Source1/RConn1
  Ideal Angular Velocity Source1/RConn2 -- Mechanical Rotational Reference1/LConn1
  Hydraulic Flow Rate Sensor1/RConn1 -- PS-Simulink Converter1/LConn1
  Fixed-Displacement Pump1/RConn1 -- Hydraulic Flow Rate Sensor1/LConn1
  Ideal Angular Velocity Source1/LConn1 -- Fixed-Displacement Pump1/LConn1

== system mysim22/Cálculo de mu ==
  Falim : Inport
  X : Inport  Port=2
  V : Inport  Port=3
  Add : Sum
  Derivative : Derivative
  Divide : Product  Inputs=*/
  Divide1 : Product  Inputs=*/
  mu : Outport
  wires:
  X/1 -> Divide/2, Derivative/1
  V/1 -> Divide1/2
  Falim/1 -> Divide1/1
  Add/1 -> mu/1  "mu ref"
  Divide/1 -> Add/1
  Derivative/1 -> Divide/1
  Divide1/1 -> Add/2

== system mysim22/Cálculo de mu1 ==
  Falim : Inport
  X : Inport  Port=2
  V : Inport  Port=3
  Add : Sum
  Derivative : Derivative
  Divide : Product  Inputs=*/
  Divide1 : Product  Inputs=*/
  mu : Outport
  wires:
  Divide1/1 -> Add/2  "D"
  Derivative/1 -> Divide/1
  Divide/1 -> Add/1  "(dX/dt)*1/X"
  Add/1 -> mu/1  "mu"
  Falim/1 -> Divide1/1
  V/1 -> Divide1/2
  X/1 -> Derivative/1, Divide/2

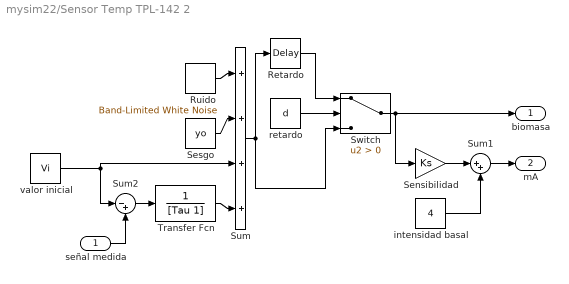
== system mysim22/Sensor Temp TPL-142 2 ==
  señal medida : Inport
  Retardo : TransportDelay  DelayTime=d
  Ruido : simulink/Sources/Band-Limited White Noise  Cov=[NP]  Ts=To  seed=[23341]
  Sensibilidad : Gain  Gain=Ks
  Sesgo : Constant  Value=yo
  Sum : Sum  Inputs=|++++  SaturateOnIntegerOverflow=on
  Sum1 : Sum  Inputs=|++
  Sum2 : Sum  Inputs=|-+
  Switch : Switch  Criteria=u2 > Threshold
  Transfer Fcn : TransferFcn  Denominator=[Tau 1]
  intensidad basal : Constant  Value=4
  retardo : Constant  Value=d
  valor inicial : Constant  Value=Vi
  biomasa : Outport
  mA : Outport  Port=2
  wires:
  Sensibilidad/1 -> Sum1/1
  Sum1/1 -> mA/1
  intensidad basal/1 -> Sum1/2
  retardo/1 -> Switch/2
  Sum/1 -> Retardo/1, Switch/3
  Retardo/1 -> Switch/1
  Switch/1 -> biomasa/1, Sensibilidad/1
  Sesgo/1 -> Sum/2
  Ruido/1 -> Sum/1
  Transfer Fcn/1 -> Sum/4
  Sum2/1 -> Transfer Fcn/1
  señal medida/1 -> Sum2/2
  valor inicial/1 -> Sum/3, Sum2/1

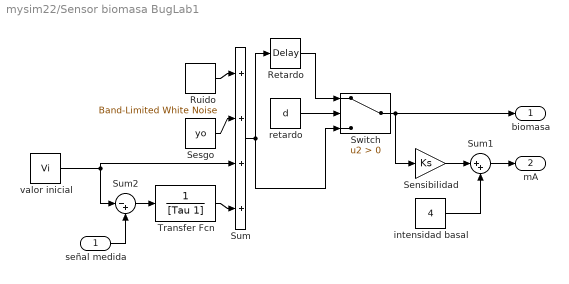
== system mysim22/Sensor biomasa BugLab1 ==
  señal medida : Inport
  Retardo : TransportDelay  DelayTime=d
  Ruido : simulink/Sources/Band-Limited White Noise  Cov=[NP]  Ts=To  seed=[23341]
  Sensibilidad : Gain  Gain=Ks
  Sesgo : Constant  Value=yo
  Sum : Sum  Inputs=|++++  SaturateOnIntegerOverflow=on
  Sum1 : Sum  Inputs=|++
  Sum2 : Sum  Inputs=|-+
  Switch : Switch  Criteria=u2 > Threshold
  Transfer Fcn : TransferFcn  Denominator=[Tau 1]
  intensidad basal : Constant  Value=4
  retardo : Constant  Value=d
  valor inicial : Constant  Value=Vi
  biomasa : Outport
  mA : Outport  Port=2
  wires:
  Sensibilidad/1 -> Sum1/1
  Sum1/1 -> mA/1
  intensidad basal/1 -> Sum1/2
  retardo/1 -> Switch/2
  Sum/1 -> Retardo/1, Switch/3
  Retardo/1 -> Switch/1
  Switch/1 -> biomasa/1, Sensibilidad/1
  Sesgo/1 -> Sum/2
  Ruido/1 -> Sum/1
  Transfer Fcn/1 -> Sum/4
  Sum2/1 -> Transfer Fcn/1
  señal medida/1 -> Sum2/2
  valor inicial/1 -> Sum/3, Sum2/1

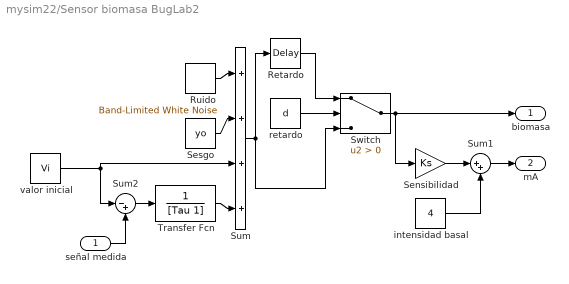
== system mysim22/Sensor biomasa BugLab2 ==
  señal medida : Inport
  Retardo : TransportDelay  DelayTime=d
  Ruido : simulink/Sources/Band-Limited White Noise  Cov=[NP]  Ts=To  seed=[23341]
  Sensibilidad : Gain  Gain=Ks
  Sesgo : Constant  Value=yo
  Sum : Sum  Inputs=|++++  SaturateOnIntegerOverflow=on
  Sum1 : Sum  Inputs=|++
  Sum2 : Sum  Inputs=|-+
  Switch : Switch  Criteria=u2 > Threshold
  Transfer Fcn : TransferFcn  Denominator=[Tau 1]
  intensidad basal : Constant  Value=4
  retardo : Constant  Value=d
  valor inicial : Constant  Value=Vi
  biomasa : Outport
  mA : Outport  Port=2
  wires:
  valor inicial/1 -> Sum2/1, Sum/3
  señal medida/1 -> Sum2/2
  Sum2/1 -> Transfer Fcn/1
  Transfer Fcn/1 -> Sum/4
  Ruido/1 -> Sum/1
  Sesgo/1 -> Sum/2
  Switch/1 -> Sensibilidad/1, biomasa/1
  Retardo/1 -> Switch/1
  Sum/1 -> Switch/3, Retardo/1
  retardo/1 -> Switch/2
  intensidad basal/1 -> Sum1/2
  Sum1/1 -> mA/1
  Sensibilidad/1 -> Sum1/1

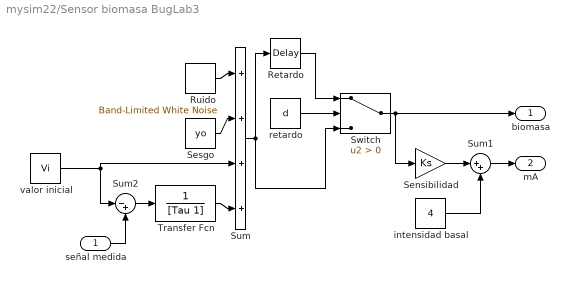
== system mysim22/Sensor biomasa BugLab3 ==
  señal medida : Inport
  Retardo : TransportDelay  DelayTime=d
  Ruido : simulink/Sources/Band-Limited White Noise  Cov=[NP]  Ts=To  seed=[23341]
  Sensibilidad : Gain  Gain=Ks
  Sesgo : Constant  Value=yo
  Sum : Sum  Inputs=|++++  SaturateOnIntegerOverflow=on
  Sum1 : Sum  Inputs=|++
  Sum2 : Sum  Inputs=|-+
  Switch : Switch  Criteria=u2 > Threshold
  Transfer Fcn : TransferFcn  Denominator=[Tau 1]
  intensidad basal : Constant  Value=4
  retardo : Constant  Value=d
  valor inicial : Constant  Value=Vi
  biomasa : Outport
  mA : Outport  Port=2
  wires:
  Sensibilidad/1 -> Sum1/1
  Sum1/1 -> mA/1
  intensidad basal/1 -> Sum1/2
  retardo/1 -> Switch/2
  Sum/1 -> Retardo/1, Switch/3
  Retardo/1 -> Switch/1
  Switch/1 -> biomasa/1, Sensibilidad/1
  Sesgo/1 -> Sum/2
  Ruido/1 -> Sum/1
  Transfer Fcn/1 -> Sum/4
  Sum2/1 -> Transfer Fcn/1
  señal medida/1 -> Sum2/2
  valor inicial/1 -> Sum/3, Sum2/1

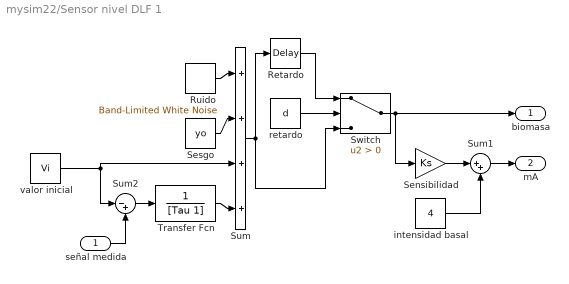
== system mysim22/Sensor nivel DLF 1 ==
  señal medida : Inport
  Retardo : TransportDelay  DelayTime=d
  Ruido : simulink/Sources/Band-Limited White Noise  Cov=[NP]  Ts=To  seed=[23341]
  Sensibilidad : Gain  Gain=Ks
  Sesgo : Constant  Value=yo
  Sum : Sum  Inputs=|++++  SaturateOnIntegerOverflow=on
  Sum1 : Sum  Inputs=|++
  Sum2 : Sum  Inputs=|-+
  Switch : Switch  Criteria=u2 > Threshold
  Transfer Fcn : TransferFcn  Denominator=[Tau 1]
  intensidad basal : Constant  Value=4
  retardo : Constant  Value=d
  valor inicial : Constant  Value=Vi
  biomasa : Outport
  mA : Outport  Port=2
  wires:
  valor inicial/1 -> Sum2/1, Sum/3
  señal medida/1 -> Sum2/2
  Sum2/1 -> Transfer Fcn/1
  Transfer Fcn/1 -> Sum/4
  Ruido/1 -> Sum/1
  Sesgo/1 -> Sum/2
  Switch/1 -> Sensibilidad/1, biomasa/1
  Retardo/1 -> Switch/1
  Sum/1 -> Switch/3, Retardo/1
  retardo/1 -> Switch/2
  intensidad basal/1 -> Sum1/2
  Sum1/1 -> mA/1
  Sensibilidad/1 -> Sum1/1

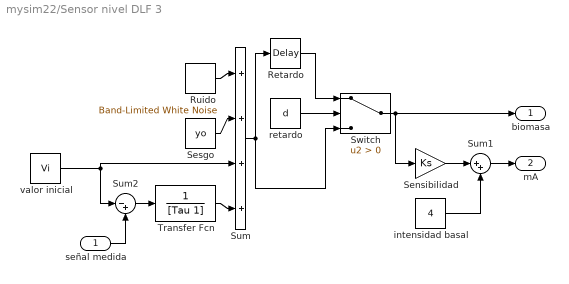
== system mysim22/Sensor nivel DLF 3 ==
  señal medida : Inport
  Retardo : TransportDelay  DelayTime=d
  Ruido : simulink/Sources/Band-Limited White Noise  Cov=[NP]  Ts=To  seed=[23341]
  Sensibilidad : Gain  Gain=Ks
  Sesgo : Constant  Value=yo
  Sum : Sum  Inputs=|++++  SaturateOnIntegerOverflow=on
  Sum1 : Sum  Inputs=|++
  Sum2 : Sum  Inputs=|-+
  Switch : Switch  Criteria=u2 > Threshold
  Transfer Fcn : TransferFcn  Denominator=[Tau 1]
  intensidad basal : Constant  Value=4
  retardo : Constant  Value=d
  valor inicial : Constant  Value=Vi
  biomasa : Outport
  mA : Outport  Port=2
  wires:
  Sensibilidad/1 -> Sum1/1
  Sum1/1 -> mA/1
  intensidad basal/1 -> Sum1/2
  retardo/1 -> Switch/2
  Sum/1 -> Retardo/1, Switch/3
  Retardo/1 -> Switch/1
  Switch/1 -> biomasa/1, Sensibilidad/1
  Sesgo/1 -> Sum/2
  Ruido/1 -> Sum/1
  Transfer Fcn/1 -> Sum/4
  Sum2/1 -> Transfer Fcn/1
  señal medida/1 -> Sum2/2
  valor inicial/1 -> Sum/3, Sum2/1

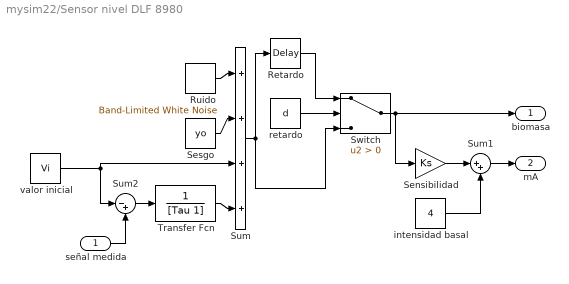
== system mysim22/Sensor nivel DLF 8980 ==
  señal medida : Inport
  Retardo : TransportDelay  DelayTime=d
  Ruido : simulink/Sources/Band-Limited White Noise  Cov=[NP]  Ts=To  seed=[23341]
  Sensibilidad : Gain  Gain=Ks
  Sesgo : Constant  Value=yo
  Sum : Sum  Inputs=|++++  SaturateOnIntegerOverflow=on
  Sum1 : Sum  Inputs=|++
  Sum2 : Sum  Inputs=|-+
  Switch : Switch  Criteria=u2 > Threshold
  Transfer Fcn : TransferFcn  Denominator=[Tau 1]
  intensidad basal : Constant  Value=4
  retardo : Constant  Value=d
  valor inicial : Constant  Value=Vi
  biomasa : Outport
  mA : Outport  Port=2
  wires:
  valor inicial/1 -> Sum2/1, Sum/3
  señal medida/1 -> Sum2/2
  Sum2/1 -> Transfer Fcn/1
  Transfer Fcn/1 -> Sum/4
  Ruido/1 -> Sum/1
  Sesgo/1 -> Sum/2
  Switch/1 -> Sensibilidad/1, biomasa/1
  Retardo/1 -> Switch/1
  Sum/1 -> Switch/3, Retardo/1
  retardo/1 -> Switch/2
  intensidad basal/1 -> Sum1/2
  Sum1/1 -> mA/1
  Sensibilidad/1 -> Sum1/1

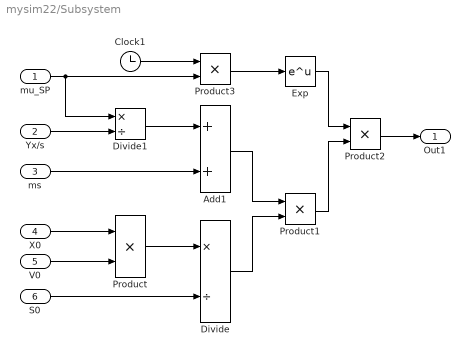
== system mysim22/Subsystem ==
  mu_SP : Inport
  Yx/s : Inport  Port=2
  ms : Inport  Port=3
  X0 : Inport  Port=4
  V0 : Inport  Port=5
  S0 : Inport  Port=6
  Add1 : Sum
  Clock1 : Clock
  Divide : Product  Inputs=*/
  Divide1 : Product  Inputs=*/
  Exp : Math  SaturateOnIntegerOverflow=on
  Product{,1..3} (4 alike) : Product
  Out1 : Outport
  wires:
  Clock1/1 -> Product3/1
  mu_SP/1 -> Divide1/1, Product3/2
  Divide/1 -> Product1/2
  Product3/1 -> Exp/1
  Add1/1 -> Product1/1
  Product/1 -> Divide/1
  Exp/1 -> Product2/1
  Product1/1 -> Product2/2
  S0/1 -> Divide/2
  Divide1/1 -> Add1/1
  Product2/1 -> Out1/1
  Yx/s/1 -> Divide1/2
  X0/1 -> Product/1
  V0/1 -> Product/2
  ms/1 -> Add1/2

== system mysim22/Subsystem1 ==
  Falim : Inport
  X : Inport  Port=2
  V : Inport  Port=3
  Cálculo de mu2 : Subsystem
  L a m2 : Gain  Gain=(4/(pi*0.337^2))/1000
  Sensor biomasa : TransferFcn  Numerator=[0.08]  Denominator=[0.0067 1]
  Sensor biomasa BugLab1 : Subsystem  Commented=on  mask{To=0.01, d=0, DS=0.075, Ks=0.08, Tau=0.0067, yo=0, Vi=0}
      mask prompts: To "Tiempo de muestreo (s)"; d "Retardo (s)"; DS "Desviacion estandar (g/L)"; Ks "Sensibilidad (mA/g/L)"; Tau "Constante de tiempo (s)"; yo "Sesgo (g/L)"; Vi "Valor inicial (g/L)"
      mask init:
      | NP=To*DS*DS;
      mask Display: image(imread('sensor_biomasa.png'))
  Sensor biomasa1 : TransferFcn  Numerator=[0.08]  Denominator=[0.033 1]
  Sensor nivel DLF 1 : Subsystem  Commented=on  mask{To=0.1, d=0, DS=0.005, Ks=0.08, Tau=0.033, yo=0, Vi=0}
      mask prompts: To "Tiempo de muestreo (s)"; d "Retardo (s)"; DS "Desviacion estandar (g/L)"; Ks "Sensibilidad (mA/g/L)"; Tau "Constante de tiempo (s)"; yo "Sesgo (g/L)"; Vi "Valor inicial (g/L)"
      mask init:
      | NP=To*DS*DS;
      mask Display: image(imread('sensor_nivel.jpg'))
  m a L2 : Gain  Gain=((pi*0.337^2)/4)*1000
  mu_ref : Outport
  wires:
  Sensor biomasa/1 -> Cálculo de mu2/2(X)  "X"
  V/1 -> L a m2/1
  m a L2/1 -> Cálculo de mu2/3(V)
  L a m2/1 -> Sensor biomasa1/1
  Sensor biomasa1/1 -> m a L2/1  "X"
  Falim/1 -> Cálculo de mu2/1(Falim)
  Cálculo de mu2/1(mu) -> mu_ref/1  "mu ref"
  X/1 -> Sensor biomasa/1

== system mysim22/Subsystem1/Cálculo de mu2 ==
  Falim : Inport
  X : Inport  Port=2
  V : Inport  Port=3
  Add : Sum
  Derivative : Derivative
  Divide : Product  Inputs=*/
  Divide1 : Product  Inputs=*/
  mu : Outport
  wires:
  X/1 -> Divide/2, Derivative/1
  V/1 -> Divide1/2
  Falim/1 -> Divide1/1
  Add/1 -> mu/1  "mu ref"
  Divide/1 -> Add/1
  Derivative/1 -> Divide/1
  Divide1/1 -> Add/2

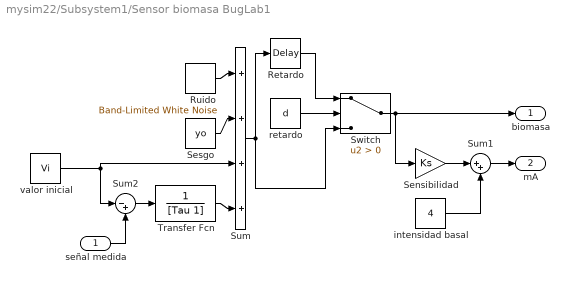
== system mysim22/Subsystem1/Sensor biomasa BugLab1 ==
  señal medida : Inport
  Retardo : TransportDelay  DelayTime=d
  Ruido : simulink/Sources/Band-Limited White Noise  Cov=[NP]  Ts=To  seed=[23341]
  Sensibilidad : Gain  Gain=Ks
  Sesgo : Constant  Value=yo
  Sum : Sum  Inputs=|++++  SaturateOnIntegerOverflow=on
  Sum1 : Sum  Inputs=|++
  Sum2 : Sum  Inputs=|-+
  Switch : Switch  Criteria=u2 > Threshold
  Transfer Fcn : TransferFcn  Denominator=[Tau 1]
  intensidad basal : Constant  Value=4
  retardo : Constant  Value=d
  valor inicial : Constant  Value=Vi
  biomasa : Outport
  mA : Outport  Port=2
  wires:
  valor inicial/1 -> Sum2/1, Sum/3
  señal medida/1 -> Sum2/2
  Sum2/1 -> Transfer Fcn/1
  Transfer Fcn/1 -> Sum/4
  Ruido/1 -> Sum/1
  Sesgo/1 -> Sum/2
  Switch/1 -> Sensibilidad/1, biomasa/1
  Retardo/1 -> Switch/1
  Sum/1 -> Switch/3, Retardo/1
  retardo/1 -> Switch/2
  intensidad basal/1 -> Sum1/2
  Sum1/1 -> mA/1
  Sensibilidad/1 -> Sum1/1

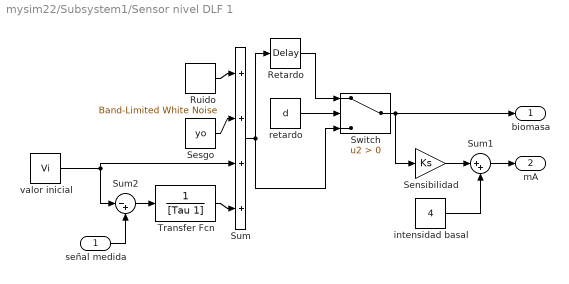
== system mysim22/Subsystem1/Sensor nivel DLF 1 ==
  señal medida : Inport
  Retardo : TransportDelay  DelayTime=d
  Ruido : simulink/Sources/Band-Limited White Noise  Cov=[NP]  Ts=To  seed=[23341]
  Sensibilidad : Gain  Gain=Ks
  Sesgo : Constant  Value=yo
  Sum : Sum  Inputs=|++++  SaturateOnIntegerOverflow=on
  Sum1 : Sum  Inputs=|++
  Sum2 : Sum  Inputs=|-+
  Switch : Switch  Criteria=u2 > Threshold
  Transfer Fcn : TransferFcn  Denominator=[Tau 1]
  intensidad basal : Constant  Value=4
  retardo : Constant  Value=d
  valor inicial : Constant  Value=Vi
  biomasa : Outport
  mA : Outport  Port=2
  wires:
  Sensibilidad/1 -> Sum1/1
  Sum1/1 -> mA/1
  intensidad basal/1 -> Sum1/2
  retardo/1 -> Switch/2
  Sum/1 -> Retardo/1, Switch/3
  Retardo/1 -> Switch/1
  Switch/1 -> biomasa/1, Sensibilidad/1
  Sesgo/1 -> Sum/2
  Ruido/1 -> Sum/1
  Transfer Fcn/1 -> Sum/4
  Sum2/1 -> Transfer Fcn/1
  señal medida/1 -> Sum2/2
  valor inicial/1 -> Sum/3, Sum2/1

== matlab function mysim22/Obs estado ==
  data: u input; y output
function y = fcn(u)
% Entradas  
Falim  = u(1); %[L/h] flujo alimentación
Fj     = u(2); %[L/h] flujo chaqueta
Tjin   = u(3); %[K] temperatura entrada chaqueta
Talim  = u(4); %[K] temperatura alimentación
Tm     = u(5); %[K] temperatura del mosto
Tj     = u(6); %[K] temperatura de la chaqueta
V      = u(7); %[L] volumen de cultivo

% Parámetros
D = Falim/V; %[h] tasa de dilución
O = 0.035;   %[g/L] concentración de saturación de oxígeno
Sin = 350;   %[g/L] concentración de glucosa en alimentación

kx1 = 0.49; %coeficiente de rendimiento de biomasa 1
kx2 = 0.05; %coeficiente de rendimiento de biomasa 2
kx3 = 0.72; %coeficiente de rendimiento de biomasa 3
ks1 = 1;    %coeficiente de rendimiento de sustrato 1
ks2 = 1;    %coeficiente de rendimiento de sustrato 2
kp2 = 0.48; %coeficiente de rendimiento de subproducto 2
kp3 = 1;    %coeficiente de rendimiento de subproducto 3

mu_s   = 3.5;                               %[gS/gX/h]
mu_o   = 0.256;                             %[gO2/gX/h]
Ks     = 0.1;                               %[gS/L]
Kip    = 10;                                %[gP/L] Kie en dewasme
Ko     = 0.0001;                            %[gO2/L]
Kp     = 0.1;                               %[gP/L] Ke en dewasme
kos    = 0.3968;                            %[gO2/gS] kos=ko1 para levadura
kop    = 1.104;                             %[gO2/gE] ko3 en dewasme
Vj     = 10;                                %[L]             
UAj    = 3750*4184*5;                       %[J/(h*K)]
rhom   = 1080;                              %[kg/m3]
rhoj   = 1000;                              %[kg/m3]  
masam  = V*rhom/1000;                       %[kg]
mf     = Falim*1.13;                        %[kg/h]
mj     = Fj;                                %[kg/h]
cpf    = 4184;                              %[J/kgK]
cpm    = 4184;                              %[J/kgK]
cpj    = 4184;                              %[J/kgK]

% Calores REVISAR UNIDADES DE TODOS
qalim  = mf*cpf*(Tm-Talim);  % alimentación [J/h]
qj     = UAj*(Tm - Tj);      % chaqueta [J/h]
qs     = 50*3600;           % agitador [J/h]
qp     = qalim + qj - qs;    % levadura [J/h]

y = [qalim qj qs qp];
